simulink model "Airshow_hotpursuit_withadjustheight"  (R2012b)
settings: Solver=ode5  StartTime=0.0  StopTime=inf  FixedStep=sample_time  RelTol=1e-3
InitFcn:
  | sample_time=0.005;%0.004;%0.0025;%0.02;
  | sample_time_Vicon = 0.005;
  | DeltaT = 0.02;
  | g = 9.81;
  | H0 = g%0.3165;
  | Kl = 1;
  | 
  | Q6_mass = 0.84;
  | 
  | Q6_Omega_r = 1.5; %for horizon ref
  | Q6_Zeta_r = 0.5; %for horizon ref
  | Q6_Omega_r_h = 2;%for vertical ref
  | Q6_Zeta_r_h = 2; %for vertical ref
  | 
  | 
  | Q6_Omega = 1.5; %for horizon control
  | Q6_Zeta = 0.5; %for horizon control
  | Q6_Omega_h= 2; %for vertical control
  | Q6_Zeta_h = 0.7; %for vertical control
  | 
  | 
  | Q6_acc_max = 5;%horizontal max acc
  | Q6_acc_max_h = 3;%horizontal max acc
  | 
  | omega_circle = 72*pi/180;
  | omega_h = 0.1;%Ascending speed
  | PI = pi;
  | Circle_R = 2.5;
  | MAX_Height = -2;
undefined symbols (not defined in the file or in its folder): DiscIntNeverNeededParam
libraries: X330_Control x5, dspswit3 x5, simulink x4
(part 2 of 4)

== matlab function Airshow_hotpursuit_withadjustheight/UAV 1/Trajectory Logic/trackbounded1 ==
  data: cpx input; cpy input; region output; cvx input; cvy input; newx output; newy output; newregion output; estsecond input; chkfinalx output; chkfinaly output; chknum output; directionflag output; distanceall output; limitspeed input; cvxy output; time input; heightcontrol output
function [region,newx,newy,newregion,chkfinalx,chkfinaly,chknum,directionflag,distanceall,cvxy,heightcontrol]  = fcn(cpx,cpy,cvx,cvy,estsecond,limitspeed,time)
%#codegen
%cp = [cpy,cpx,0];
%cpest = [estrawy, estrawx,0];
%%database of check points
if(time<1)
    cvxy = 0;
else
cvxy = sqrt(cvx^2 + cvy^2);
end
chk0x = 3.239;
chk0y = 0.7037;
chk1x = 2.598;
chk1y = 1.13;
chk2x = 1.853;
chk2y = 1.266;
chk3x = 1.124;
chk3y = 1.462;
chk4x = 0.39;
chk4y = 1.935;
chk5x = -0.393;
chk5y = 2.012;
chk6x = -1.038;
chk6y = 1.521;
chk7x = -1.644;
chk7y = 1.023;
chk8x = -2.269;
chk8y = 1.058;
chk9x = -2.847;
chk9y = 1.469;
chk10x = -3.795;
chk10y = 1.337;
chk11x = -3.985;
chk11y = 0.42;
chk12x = -3.844;
chk12y = -0.55;
chk13x = -3.363;
chk13y = -1.263;
chk14x = -2.592;
chk14y = -1.786;
chk15x = -1.645;
chk15y = -2.067;
chk16x = -0.5438;
chk16y = -2.227;
chk17x = 0.425;
chk17y = -2.141;
chk18x = 1.192;
chk18y = -1.755;
chk19x = 2.025;
chk19y = -1.113;
chk20x = 3.12;
chk20y = -0.9148;
%%%%%%%%%%%%%%%%%%%%%%%%%%%%%%%%%%%%%%%%%%%%%%%%%%%%%%%%%%%
chk0 = [chk0y,chk0x,0];
chk1 = [chk1y,chk1x,0];
chk2 = [chk2y,chk2x,0];
chk3 = [chk3y,chk3x,0];
chk4 = [chk4y,chk4x,0];
chk5 = [chk5y,chk5x,0];
chk6 = [chk6y,chk6x,0];
chk7 = [chk7y,chk7x,0];
chk8 = [chk8y,chk8x,0];
chk9 = [chk9y,chk9x,0];
chk10 = [chk10y,chk10x,0];
chk11 = [chk11y,chk11x,0];
chk12 = [chk12y,chk12x,0];
chk13 = [chk13y,chk13x,0];
chk14 = [chk14y,chk14x,0];
chk15 = [chk15y,chk15x,0];
chk16 = [chk16y,chk16x,0];
chk17 = [chk17y,chk17x,0];
chk18 = [chk18y,chk18x,0];
chk19 = [chk19y,chk19x,0];
chk20 = [chk20y,chk20x,0];


distance01 = sqrt((chk0y-chk1y)^2+(chk0x-chk1x)^2);
distance12 = sqrt((chk2y-chk1y)^2+(chk2x-chk1x)^2);
distance23 = sqrt((chk2y-chk3y)^2+(chk2x-chk3x)^2);
distance34 = sqrt((chk3y-chk4y)^2+(chk3x-chk4x)^2);
distance45 = sqrt((chk4y-chk5y)^2+(chk4x-chk5x)^2);
distance56 = sqrt((chk5y-chk6y)^2+(chk5x-chk6x)^2);
distance67 = sqrt((chk6y-chk7y)^2+(chk6x-chk7x)^2);
distance78 = sqrt((chk7y-chk8y)^2+(chk7x-chk8x)^2);
distance89 = sqrt((chk8y-chk9y)^2+(chk8x-chk9x)^2);
distance910 = sqrt((chk9y-chk10y)^2+(chk9x-chk10x)^2);
distance1011 = sqrt((chk10y-chk11y)^2+(chk10x-chk11x)^2);
distance1112 = sqrt((chk11y-chk12y)^2+(chk11x-chk12x)^2);
distance1213 = sqrt((chk12y-chk13y)^2+(chk12x-chk13x)^2);
distance1314 = sqrt((chk13y-chk14y)^2+(chk13x-chk14x)^2);
distance1415 = sqrt((chk14y-chk15y)^2+(chk14x-chk15x)^2);
distance1516 = sqrt((chk15y-chk16y)^2+(chk15x-chk16x)^2);
distance1617 = sqrt((chk16y-chk17y)^2+(chk16x-chk17x)^2);
distance1718 = sqrt((chk17y-chk18y)^2+(chk17x-chk18x)^2);
distance1819 = sqrt((chk18y-chk19y)^2+(chk18x-chk19x)^2);
distance1920 = sqrt((chk19y-chk20y)^2+(chk19x-chk20x)^2);
distance200 = sqrt((chk20y-chk0y)^2+(chk20x-chk0x)^2);
distanceall = distance01 + distance12 + distance23+distance34+distance45+distance56+distance67+distance78+distance89+distance910+distance1011+distance1112+distance1213+distance1314+distance1415+distance1516+distance1617+distance1718+distance1819+distance1920+distance200;
%%%%%%%%%%%%%%%%%%%%%%%%%%%%%%%%%%%%%%%%%%%%%%%%%%%%%%%%%%%%%%%%%%%%%%%%%%%%%%%%%%%%%%region selector
if(cpx>-5 && cpx<=-4 && cpy>-3 && cpy<=-2)
    region = 0;
elseif(cpx>-4 && cpx<=-3 && cpy>-3 && cpy<=-2 )
    region = 1;
elseif(cpx>-3 && cpx<=-2 && cpy>-3 && cpy<=-2 )
    region = 2;
elseif(cpx>-2 && cpx<=-1 && cpy>-3 &&cpy<=-2)
    region = 3;
elseif(cpx>-1 && cpx<=0 && cpy>-3 && cpy<=-2)
    region = 4;
elseif(cpx>0 && cpx<=1 &&cpy>-3 && cpy<=-2)
    region = 5;
elseif(cpx>1 && cpx<=2 && cpy>-3 && cpy<=-2)
    region = 6;
elseif(cpx>2 && cpx<=3 && cpy>-3 && cpy<=-2)
    region = 7;
elseif(cpx>3 && cpx<=4 && cpy>-3 && cpy<=-2)
    region = 8;
elseif(cpx>4&& cpx<=5 && cpy>-3 && cpy<=-2)
    region = 9;
elseif(cpx>-5 && cpx<=-4 && cpy>-2 && cpy<=-1)
    region = 10;
elseif(cpx>-4 && cpx<=-3 && cpy>-2 && cpy<=-1)
    region = 11;
elseif(cpx>-3 && cpx<=-2 && cpy>-2 && cpy<=-1)
    region = 12;
elseif(cpx>-2 && cpx<=-1 && cpy>-2 && cpy<=-1)
    region = 13;
elseif(cpx>-1 && cpx<=0 && cpy>-2 && cpy<=-1)
    region = 14;
elseif(cpx>0 && cpx<=1 && cpy>-2 && cpy<=-1)
    region = 15;
elseif(cpx>1 && cpx<=2 && cpy>-2 && cpy<=-1)
    region = 16;
elseif(cpx>2 && cpx<=3 && cpy>-2 && cpy<=-1)
    region = 17;
elseif(cpx>3 && cpx<=4 && cpy>-2 && cpy<=-1)
    region = 18;
elseif(cpx>4 && cpx<=5 && cpy>-2 && cpy<=-1)
    region = 19;
elseif(cpx>-5 && cpx<=-4 && cpy>-1 && cpy<=0)
    region = 20;
elseif(cpx>-4 && cpx<=-3 && cpy>-1 && cpy<=0)
    region = 21;
elseif(cpx>-3 && cpx<=-2 && cpy>-1 && cpy<=0)
    region = 22;
elseif(cpx>-2 && cpx<=-1 && cpy>-1 && cpy<=0)
    region = 23;
elseif(cpx>-1 && cpx<=0 && cpy>-1 && cpy<=0)
    region = 24;
elseif(cpx>0 && cpx<=1 && cpy>-1 && cpy<=0)
    region = 25;
elseif(cpx>1 && cpx<=2 && cpy>-1 && cpy<=0)
    region = 26;
elseif(cpx>2 && cpx<=3 && cpy>-1 && cpy<=0)
    region = 27;
elseif(cpx>3 && cpx<=4 && cpy>-1 && cpy<=0)
    region = 28;
elseif(cpx>4 && cpx<=5 && cpy>-1 && cpy<=0)
    region = 29;
elseif(cpx>-5 && cpx<=-4 && cpy>0 && cpy<=1)
    region = 30;
elseif(cpx>-4 && cpx<=-3 && cpy>0 && cpy<=1)
    region = 31;
elseif(cpx>-3 && cpx<=-2 && cpy>0 && cpy<=1)
    region = 32;
elseif(cpx>-2 && cpx<=-1 && cpy>0 && cpy<=1)
    region = 33;
elseif(cpx>-1 && cpx<=0 && cpy>0 && cpy<=1)
    region = 34;
elseif(cpx>0 && cpx<=1 && cpy>0 && cpy<=1)
    region = 35;
elseif(cpx>1 && cpx<=2 && cpy>0 && cpy<=1)
    region = 36;
elseif(cpx>2 && cpx<=3 && cpy>0 && cpy<=1)
    region = 37;
elseif(cpx>3 && cpx<=4 && cpy>0 && cpy<=1)
    region = 38;
elseif(cpx>4 && cpx<=5 && cpy>0 && cpy<=1)
    region = 39;
elseif(cpx>-5 && cpx<=-4 && cpy>1 && cpy<=2)
    region = 40;
elseif(cpx>-4 && cpx<=-3 && cpy>1 && cpy<=2)
    region = 41;
elseif(cpx>-3 && cpx<=-2&& cpy>1 && cpy<=2)
    region = 42;
elseif(cpx>-2 && cpx<=-1 && cpy>1 && cpy<=2)
    region = 43;
elseif(cpx>-1 && cpx<=0 && cpy>1 && cpy<=2)
    region = 44;
elseif(cpx>0 && cpx<=1 && cpy>1 && cpy<=2)
    region = 45;
elseif(cpx>1 && cpx<=2 && cpy>1 && cpy<=2)
    region = 46;
elseif(cpx>2 && cpx<=3 && cpy>1 && cpy<=2)
    region = 47;
elseif(cpx>3 && cpx<=4 && cpy>1 && cpy<=2)
    region = 48;
elseif(cpx>4 && cpx<=5 && cpy>1 && cpy<=2)
    region = 49;
elseif(cpx>-5 && cpx<=-4 && cpy>2 && cpy<=3)
    region = 50;
elseif(cpx>-4 && cpx<=-3 && cpy>2 && cpy<=3)
    region = 51;
elseif(cpx>-3 && cpx<=-2 && cpy>2 && cpy<=3)
    region = 52;
elseif(cpx>-2 && cpx<=-1 && cpy>2 && cpy<=3)
    region = 53;
elseif(cpx>-1 && cpx<=0 && cpy>2 && cpy<=3)
    region = 54;
elseif(cpx>0 && cpx<=1 && cpy>2 && cpy<=3)
    region = 55;
elseif(cpx>1 && cpx<=2 && cpy>2 && cpy<=3)
    region = 56;
elseif(cpx>2 && cpx<=3 && cpy>2 && cpy<=3)
    region = 57;
elseif(cpx>3 && cpx<=4 && cpy>2 && cpy<=3)
    region = 58;
elseif(cpx>4 && cpx<=5 && cpy>2 && cpy<=3)
    region = 59;
else
    region = -1;
end
%%%%%%%%%%%%%%%%%%%%%%%%%%%%%%%%%%%%%%%%%%%%%%%%%%%%%%%%%%%%%%%%%%%%%%%%%%%%%%%%%%%%%%%%%%%%%%%%%%
if(region==37 ||region==48)
    %%%%%%%%%%%%%%%%calculate point to line distance%%%%%%%%%%%
    %a = chk1 - chk0;
   % b = cp - chk0;
    %d = norm(cross(a,b)) / norm(a);
    angle = atan2((chk1x-chk0x),(chk1y-chk0y));
    samplex = chk0x;
    sampley = chk0y;
    zero = 1;

elseif(region == 36||region==47)
    %a = chk2 - chk1;
   % b = cp - chk1;
   % d = norm(cross(a,b)) / norm(a);
    angle = atan2((chk2x-chk1x),(chk2y-chk1y));
    zero = 1;
    samplex = chk1x;
    sampley = chk1y;
elseif(region == 46 ||region==56)
    %a = chk3 - chk2;
    %b = cp - chk2;
   % d = norm(cross(a,b)) / norm(a);
    angle = atan2((chk3x-chk2x),(chk3y-chk2y));
    zero = 1;
    samplex = chk2x;
    sampley = chk2y;
elseif(region == 45 || region==55 ||region==35)
   % a = chk4 - chk3;
   % b = cp - chk3;
    %d = norm(cross(a,b)) / norm(a);
    angle = atan2((chk4x-chk3x),(chk4y-chk3y));
    zero = 1;
      samplex = chk3x;
    sampley = chk3y;
elseif(region == 54||region==44)
    %a = chk5 - chk4;
    %b = cp - chk4;
    %d = norm(cross(a,b)) / norm(a);
    angle = atan2((chk5x-chk4x),(chk5y-chk4y));
    zero = 1;
    samplex = chk4x;
    sampley = chk4y;
elseif(region == 43||region==53)
    %a = chk6 - chk5;
    %b = cp - chk5;
    %d = norm(cross(a,b)) / norm(a);
    angle = atan2((chk6x-chk5x),(chk6y-chk5y));
    zero = 1;
    samplex = chk5x;
    sampley = chk5y;
elseif(region==33||region==34)
    %a = chk7 - chk6;
    %b = cp - chk6;
    %d = norm(cross(a,b)) / norm(a);
    angle = atan2((chk7x-chk6x),(chk7y-chk6y));
    zero = 1;
    samplex = chk6x;
    sampley = chk6y;
elseif(region == 32)
    %a = chk8 - chk7;
    %b = cp - chk7;
    %d = norm(cross(a,b)) / norm(a);
    angle = atan2((chk8x-chk7x),(chk8y-chk7y));
    zero = 1;
    samplex = chk7x;
    sampley = chk7y;
elseif(region==42)
    %a = chk9 - chk8;
    %b = cp - chk8;
    %d = norm(cross(a,b)) / norm(a);
    angle = atan2((chk9x-chk8x),(chk9y-chk8y));
    zero = 1;
    samplex = chk8x;
    sampley = chk8y;
elseif(region == 41||region==31)
    %a = chk10 - chk9;
    %b = cp - chk9;
    %d = norm(cross(a,b)) / norm(a);
    angle = atan2((chk10x-chk9x),(chk10y-chk9y));
    zero = 1;
    samplex = chk9x;
    sampley = chk9y;
elseif(region == 30||region==40)
    %a = chk11 - chk10;
    %b = cp - chk10;
    %d = norm(cross(a,b)) / norm(a);
    angle = atan2((chk11x-chk10x),(chk11y-chk10y));
    zero = 1;
    samplex = chk10x;
    sampley = chk10y;
elseif(region == 20||region==21)
    %a = chk12 - chk11;
    %b = cp - chk11;
    %d = norm(cross(a,b)) / norm(a);
    angle = atan2((chk12x-chk11x),(chk12y-chk11y));
    zero = 1;
    samplex = chk11x;
    sampley = chk11y;
elseif(region == 10||region==11)
    %a = chk13 - chk12;
    %b = cp - chk12;
    %d = norm(cross(a,b)) / norm(a);
    angle = atan2((chk13x-chk12x),(chk13y-chk12y));
    zero = 1;
    samplex = chk12x;
    sampley = chk12y;
elseif(region == 1||region==12)
    %a = chk14 - chk13;
    %b = cp - chk13;
    %d = norm(cross(a,b)) / norm(a);
    angle = atan2((chk14x-chk13x),(chk14y-chk13y));
    zero = 1;
    samplex = chk13x;
    sampley = chk13y;
elseif(region == 2||region==13)
    %a = chk15 - chk14;
    %b = cp - chk14;
    %d = norm(cross(a,b)) / norm(a);
    angle = atan2((chk15x-chk14x),(chk15y-chk14y));
    zero = 1;
    samplex = chk14x;
    sampley = chk14y;
elseif(region == 3||region==14)
    %a = chk16 - chk15;
    %b = cp - chk15;
    %d = norm(cross(a,b)) / norm(a);
    angle = atan2((chk16x-chk15x),(chk16y-chk15y));
    zero = 1;
    samplex = chk15x;
    sampley = chk15y;
elseif(region == 4||region==5)
    %a = chk17 - chk16;
    %b = cp - chk16;
    %d = norm(cross(a,b)) / norm(a);
    angle = atan2((chk17x-chk16x),(chk17y-chk16y));
    zero = 1;
    samplex = chk16x;
    sampley = chk16y;
elseif(region == 6||region==15)
    %a = chk18 - chk17;
    %b = cp - chk17;
    %d = norm(cross(a,b)) / norm(a);
    angle = atan2((chk18x-chk17x),(chk18y-chk17y));
    zero = 1;
    samplex = chk17x;
    sampley = chk17y;
elseif(region == 16||region==7||region==25)
    %a = chk19 - chk18;
    %b = cp - chk18;
    %d = norm(cross(a,b)) / norm(a);
    angle = atan2((chk19x-chk18x),(chk19y-chk18y));
    zero = 1;
    samplex = chk18x;
    sampley = chk18y;
elseif(region == 26||region==27||region == 17 || region == 18)%%%%%%%%%%%%%%%%%%%%%%%%%%%%%%%%%%%%%%%%%%%%%%%%need to test
    %a = chk20 - chk19;
    %b = cp - chk19;
    %d = norm(cross(a,b)) / norm(a);
    angle = atan2((chk20x-chk19x),(chk20y-chk19y));
    zero = 1;
    samplex = chk19x;
    sampley = chk19y;
elseif(region == 28||region==29||region == 38 || region == 39) %%need to test 6 feb
    %a = chk0 - chk20;
    %b = cp - chk20;
    %d = norm(cross(a,b)) / norm(a);
    angle = atan2((chk0x-chk20x),(chk0y-chk20y));
    zero = 1;
    samplex = chk20x;
    sampley = chk20y;
else
    %a = -1;
   % b = -1;
    %d = -1;
    angle = -1;%%% i know this is not correct i will add one more zero coefficient to cancel this case
    zero = 0;
    samplex = 0;
    sampley = 0;
end


%%%%%%%%%%%%%%%%%%%%%%%%%%%%%%%%%%%%%%%%%%%%%%%%%%%%%%%%%%%%%%%%%%%%%%%%%%%%%%%%%%%%%%%%%%%%%%%%%%
% %%calculate project point on the check point line
if(zero == 0)%%if out of boundary none of the region match
        newy = 100;
        newx = 100;
else   %%match the region

        if(angle == 0 ||angle == 180)
            newx  = samplex;
            newy = cpy;
        elseif(angle == 90 || angle == 270)
            newx = cpx;
            newy = sampley;
        else
         kk = -1/(tan(angle));
         m = cpx - kk*cpy ;
         k = tan(angle);
         newy = (samplex - k*sampley - m)/(kk - k);
         newx = kk*newy + m;
         end

end

if(newx>-5 && newx<=-4 && newy>-3 && newy<=-2)
    newregion = 0;
elseif(newx>-4 && newx<=-3 && newy>-3 && newy<=-2 )
    newregion = 1;
elseif(newx>-3 && newx<=-2 && newy>-3 && newy<=-2 )
    newregion = 2;
elseif(newx>-2 && newx<=-1 && newy>-3 &&newy<=-2)
    newregion = 3;
elseif(newx>-1 && newx<=0 && newy>-3 && newy<=-2)
    newregion = 4;
elseif(newx>0 && newx<=1 &&newy>-3 && newy<=-2)
    newregion = 5;
elseif(newx>1 && newx<=2 && newy>-3 && newy<=-2)
    newregion = 6;
elseif(newx>2 && newx<=3 && newy>-3 && newy<=-2)
    newregion = 7;
elseif(newx>3 && newx<=4 && newy>-3 && newy<=-2)
    newregion = 8;
elseif(newx>4&& newx<=5 && newy>-3 && newy<=-2)
    newregion = 9;
elseif(newx>-5 && newx<=-4 && newy>-2 && newy<=-1)
    newregion = 10;
elseif(newx>-4 && newx<=-3 && newy>-2 && newy<=-1)
    newregion = 11;
elseif(newx>-3 && newx<=-2 && newy>-2 && newy<=-1)
    newregion = 12;
elseif(newx>-2 && newx<=-1 && newy>-2 && newy<=-1)
    newregion = 13;
elseif(newx>-1 && newx<=0 && newy>-2 && newy<=-1)
    newregion = 14;
elseif(newx>0 && newx<=1 && newy>-2 && newy<=-1)
    newregion = 15;
elseif(newx>1 && newx<=2 && newy>-2 && newy<=-1)
    newregion = 16;
elseif(newx>2 && newx<=3 && newy>-2 && newy<=-1)
    newregion = 17;
elseif(newx>3 && newx<=4 && newy>-2 && newy<=-1)
    newregion = 18;
elseif(newx>4 && newx<=5 && newy>-2 && newy<=-1)
    newregion = 19;
elseif(newx>-5 && newx<=-4 && newy>-1 && newy<=0)
    newregion = 20;
elseif(newx>-4 && newx<=-3 && newy>-1 && newy<=0)
    newregion = 21;
elseif(newx>-3 && newx<=-2 && newy>-1 && newy<=0)
    newregion = 22;
elseif(newx>-2 && newx<=-1 && newy>-1 && newy<=0)
    newregion = 23;
elseif(newx>-1 && newx<=0 && newy>-1 && newy<=0)
    newregion = 24;
elseif(newx>0 && newx<=1 && newy>-1 && newy<=0)
    newregion = 25;
elseif(newx>1 && newx<=2 && newy>-1 && newy<=0)
    newregion = 26;
elseif(newx>2 && newx<=3 && newy>-1 && newy<=0)
    newregion = 27;
elseif(newx>3 && newx<=4 && newy>-1 && newy<=0)
    newregion = 28;
elseif(newx>4 && newx<=5 && newy>-1 && newy<=0)
    newregion = 29;
elseif(newx>-5 && newx<=-4 && newy>0 && newy<=1)
    newregion = 30;
elseif(newx>-4 && newx<=-3 && newy>0 && newy<=1)
    newregion = 31;
elseif(newx>-3 && newx<=-2 && newy>0 && newy<=1)
    newregion = 32;
elseif(newx>-2 && newx<=-1 && newy>0 && newy<=1)
    newregion = 33;
elseif(newx>-1 && newx<=0 && newy>0 && newy<=1)
    newregion = 34;
elseif(newx>0 && newx<=1 && newy>0 && newy<=1)
    newregion = 35;
elseif(newx>1 && newx<=2 && newy>0 && newy<=1)
    newregion = 36;
elseif(newx>2 && newx<=3 && newy>0 && newy<=1)
    newregion = 37;
elseif(newx>3 && newx<=4 && newy>0 && newy<=1)
    newregion = 38;
elseif(newx>4 && newx<=5 && newy>0 && newy<=1)
    newregion = 39;
elseif(newx>-5 && newx<=-4 && newy>1 && newy<=2)
    newregion = 40;
elseif(newx>-4 && newx<=-3 && newy>1 && newy<=2)
    newregion = 41;
elseif(newx>-3 && newx<=-2&& newy>1 && newy<=2)
    newregion = 42;
elseif(newx>-2 && newx<=-1 && newy>1 && newy<=2)
    newregion = 43;
elseif(newx>-1 && newx<=0 && newy>1 && newy<=2)
    newregion = 44;
elseif(newx>0 && newx<=1 && newy>1 && newy<=2)
    newregion = 45;
elseif(newx>1 && newx<=2 && newy>1 && newy<=2)
    newregion = 46;
elseif(newx>2 && newx<=3 && newy>1 && newy<=2)
    newregion = 47;
elseif(newx>3 && newx<=4 && newy>1 && newy<=2)
    newregion = 48;
elseif(newx>4 && newx<=5 && newy>1 && newy<=2)
    newregion = 49;
elseif(newx>-5 && newx<=-4 && newy>2 && newy<=3)
    newregion = 50;
elseif(newx>-4 && newx<=-3 && newy>2 && newy<=3)
    newregion = 51;
elseif(newx>-3 && newx<=-2 && newy>2 && newy<=3)
    newregion = 52;
elseif(newx>-2 && newx<=-1 && newy>2 && newy<=3)
    newregion = 53;
elseif(newx>-1 && newx<=0 && newy>2 && newy<=3)
    newregion = 54;
elseif(newx>0 && newx<=1 && newy>2 && newy<=3)
    newregion = 55;
elseif(newx>1 && newx<=2 && newy>2 && newy<=3)
    newregion = 56;
elseif(newx>2 && newx<=3 && newy>2 && newy<=3)
    newregion = 57;
elseif(newx>3 && newx<=4 && newy>2 && newy<=3)
    newregion = 58;
elseif(newx>4 && newx<=5 && newy>2 && newy<=3)
    newregion = 59;
else
    newregion = -1;
end

%%%%%%%%%%%%%%%%%%%%%%%%%%%%%%%%%%%%%%%%%%%%%%%%%%%%%%%%%%%%%%%%%%%%%%%%%%%%
% if(posx>-2 && posx<=-1 && posy>1 && posy<=2)
%     posregion = 0;
% elseif(posx>-1 && posx<=0 && posy>1 && posy<=2 )
%     posregion = 1;
% elseif(posx>0 && posx<=1 && posy>1 && posy<=2 )
%     posregion = 2;
% elseif(posx>-2 && posx<=-1 && posy>0 &&posy<=1)
%     posregion = 3;
% elseif(posx>-1 && posx<=0 && posy>0 && posy<=1)
%     posregion = 4;
% elseif(posx>-2 && posx<=-1 &&posy>-1 && posy<=0)
%     posregion = 5;
% elseif(posx>-1 && posx<=0 && posy>-1 && posy<=0)
%     posregion = 6;
% elseif(posx>-2 && posx<=-1 && posy>-2 && posy<=-1)
%     posregion = 7;
% elseif(posx>-1 && posx<=0 && posy>-2 && posy<=-1)
%     posregion = 8;
% elseif(posx>0 && posx<=1 && posy>-2 && posy<=-1)
%     posregion = 9;
% elseif(posx>1 && posx<=2 && posy>-2 && posy<=-1)
%     posregion = 10;
% elseif(posx>0 && posx<=1 && posy>-1 && posy<=0)
%     posregion = 11;
% elseif(posx>1 && posx<=2 && posy>-1 && posy<=0)
%     posregion = 12;
% elseif(posx>1 && posx<=2 && posy>0 && posy<=1)
%     posregion = 13;
% elseif(posx>1 && posx<=2 && posy>1 && posy<=2)
%     posregion = 14;
% elseif(posx>0 && posx<=1 && posy>0 && posy<=1)
%     posregion = 15;
% elseif(posx>2 && posx<=3 && posy>-2 && posy<=-1)
%     posregion = 16;
% elseif(posx>1 && posx<=2 && posy>-3 && posy<=-2)
%     posregion = 17;
% elseif(posx>2 && posx<=3 && posy>-3 && posy<=-2)
%     posregion = 18;
% elseif(posx>0 && posx<=1 && posy>-3 && posy<=-2)
%     posregion = 19;
% elseif(posx>-1 && posx<=0 && posy>-3 && posy<=-2)
%     posregion = 20;
% elseif(posx>2 && posx<=3 && posy>-1 && posy<=0)
%     posregion = 21;
% elseif(posx>2 && posx<=3 && posy>0 && posy<=1)
%     posregion = 22;
% elseif(posx>1 && posx<=2 && posy>2 && posy<=3)
%     posregion = 23;
% elseif(posx>0 && posx<=1 && posy>2 && posy<=3)
%    posregion = 24;
% elseif(posx>-1 && posx<=0 && posy>2 && posy<=3)
%     posregion = 25;
% else
%     posregion = -1;
% end


%%%%%%%%%%%%%%%%%%%%%%%%%%%%%%%%%%%%%%%%%%%%%%%%%%%%%%%%%%%%%%%%%%%%%%%%%
velangle = atan2(cvx,cvy);
diffvelangletoangle = velangle - angle;
velproject = (cvx^2 + cvy^2)*cos(diffvelangletoangle);
estdistance = estsecond * velproject;
vxyM = sqrt(cvx^2 + cvy^2);
cosdiffvelangletoangle = cos(diffvelangletoangle);
if(vxyM < limitspeed)
    directionflag = 0;
    %frontbackflag = -1;
    %diffuavcartoangle = -9999;
else
if(cosdiffvelangletoangle>=0)
    directionflag = 1;
else
    directionflag = -1;
end
%uavcarvectorangle = atan2((posx-newx),(posy-newy));
%diffuavcartoangle = uavcarvectorangle - angle;
% cosdiffuavcartoangle = cos(diffuavcartoangle);
% if(cosdiffuavcartoangle>=0)
%     frontbackflag = 1;
% else
%     frontbackflag = 0;
% end
end
%if(directionflag == 1)
if(newregion == 48 ||newregion==37)
    newdistancetonext = sqrt((newy-chk1y)^2+(newx-chk1x)^2);
    if(estdistance < (newdistancetonext))
        chkfinalx = chk1x;
        chkfinaly = chk1y;
        chknum = 1;
    elseif(estdistance>=(newdistancetonext) && estdistance <((newdistancetonext) + distance12))
        chkfinalx = chk2x;
        chkfinaly = chk2y;
        chknum = 2;
    elseif(estdistance>=((newdistancetonext)+distance12)&&estdistance<((newdistancetonext)+distance12+distance23))
        chkfinalx = chk3x;
        chkfinaly = chk3y;
        chknum = 3;
    elseif(estdistance>=((newdistancetonext)+distance12+distance23)&&estdistance<((newdistancetonext)+distance12+distance23+distance34))
        chkfinalx = chk4x;
        chkfinaly = chk4y;
        chknum = 4;
    elseif(estdistance>=((newdistancetonext)+distance12+distance23+distance34)&&estdistance<((newdistancetonext)+distance12+distance23+distance34+distance45))
        chkfinalx = chk5x;
        chkfinaly = chk5y;
        chknum = 5;
    else
        chkfinalx = chk5x;
        chkfinaly = chk5y;
        chknum = 5;
    end
elseif(newregion == 36||newregion==47)
    newdistancetonext = sqrt((newy-chk2y)^2+(newx-chk2x)^2);
    if(estdistance < (newdistancetonext))
        chkfinalx = chk2x;
        chkfinaly = chk2y;
        chknum = 2;
    elseif(estdistance >=(newdistancetonext)&&estdistance < ((newdistancetonext)+distance23))
        chkfinalx = chk3x;
        chkfinaly = chk3y;
        chknum = 3;
    elseif(estdistance >=((newdistancetonext)+distance23)&&estdistance < ((newdistancetonext)+distance23+distance34))
        chkfinalx = chk4x;
        chkfinaly = chk4y;
        chknum = 4;
    elseif(estdistance >=((newdistancetonext)+distance23+distance34)&&estdistance < ((newdistancetonext)+distance23+distance34+distance45))
        chkfinalx = chk5x;
        chkfinaly = chk5y;
        chknum = 5;
    elseif(estdistance >=((newdistancetonext)+distance23+distance34+distance45)&&estdistance < ((newdistancetonext)+distance23+distance34+distance45+distance56))
        chkfinalx = chk6x;
        chkfinaly = chk6y;
        chknum = 6;
    else
        chkfinalx = chk6x;
        chkfinaly = chk6y;
        chknum = 6;
    end
elseif(newregion == 46||newregion==56)
    newdistancetonext = sqrt((newy-chk3y)^2+(newx-chk3x)^2);
    if(estdistance < (newdistancetonext))
        chkfinalx = chk3x;
        chkfinaly = chk3y;
        chknum = 3;
    elseif((estdistance >= (newdistancetonext))&&estdistance<((newdistancetonext)+distance34))
        chkfinalx = chk4x;
        chkfinaly = chk4y;
        chknum = 4;
    elseif((estdistance >= (newdistancetonext)+distance34)&&estdistance<((newdistancetonext)+distance34+distance45))
        chkfinalx = chk5x;
        chkfinaly = chk5y;
        chknum = 5;
    elseif((estdistance >= (newdistancetonext)+distance34+distance45)&&estdistance<((newdistancetonext)+distance34+distance45+distance56))
        chkfinalx = chk6x;
        chkfinaly = chk6y;
        chknum = 6;
    elseif((estdistance >= (newdistancetonext)+distance34+distance45+distance56)&&estdistance<((newdistancetonext)+distance34+distance45+distance56+distance67))
        chkfinalx = chk7x;
        chkfinaly = chk7y;
        chknum = 7;
    else
        chkfinalx = chk7x;
        chkfinaly = chk7y;
        chknum = 7;
    end
elseif(newregion ==45 || newregion == 55|| newregion == 35)
    newdistancetonext = sqrt((newy-chk4y)^2+(newx-chk4x)^2);
    if(estdistance < (newdistancetonext))
        chkfinalx = chk4x;
        chkfinaly = chk4y;
        chknum = 4;
    elseif((estdistance >= (newdistancetonext))&&estdistance<((newdistancetonext)+distance45))
        chkfinalx = chk5x;
        chkfinaly = chk5y;
        chknum = 5;
    elseif((estdistance >= (newdistancetonext)+distance45)&&estdistance<((newdistancetonext)+distance45+distance56))
        chkfinalx = chk6x;
        chkfinaly = chk6y;
        chknum = 6;
    elseif((estdistance >= (newdistancetonext)+distance45+distance56)&&estdistance<((newdistancetonext)+distance45+distance56+distance67))
        chkfinalx = chk7x;
        chkfinaly = chk7y;
        chknum = 7;
    elseif((estdistance >= (newdistancetonext)+distance45+distance56+distance67)&&estdistance<((newdistancetonext)+distance45+distance56+distance67+distance78))
        chkfinalx = chk8x;
        chkfinaly = chk8y;
        chknum = 8;
    else
        chkfinalx = chk8x;
        chkfinaly = chk8y;
        chknum = 8;
    end
elseif(newregion == 54|| newregion == 44)
    newdistancetonext = sqrt((newy-chk5y)^2+(newx-chk5x)^2);
    if(estdistance < (newdistancetonext))
        chkfinalx = chk5x;
        chkfinaly = chk5y;
        chknum = 5;
    elseif((estdistance >= (newdistancetonext))&&estdistance<((newdistancetonext)+distance56))
        chkfinalx = chk6x;
        chkfinaly = chk6y;
        chknum = 6;
    elseif((estdistance >= (newdistancetonext)+distance56)&&estdistance<((newdistancetonext)+distance56+distance67))
        chkfinalx = chk7x;
        chkfinaly = chk7y;
        chknum = 7;
    elseif((estdistance >= (newdistancetonext)+distance56+distance67)&&estdistance<((newdistancetonext)+distance56+distance67+distance78))
        chkfinalx = chk8x;
        chkfinaly = chk8y;
        chknum = 8;
    elseif((estdistance >= (newdistancetonext)+distance56+distance67+distance78)&&estdistance<((newdistancetonext)+distance56+distance67+distance78+distance89))
        chkfinalx = chk9x;
        chkfinaly = chk9y;
        chknum = 9;
    else
        chkfinalx = chk9x;
        chkfinaly = chk9y;
        chknum = 9;
    end
elseif(newregion == 43|| newregion == 53)
    newdistancetonext = sqrt((newy-chk6y)^2+(newx-chk6x)^2);
    if(estdistance < (newdistancetonext))
        chkfinalx = chk6x;
        chkfinaly = chk6y;
        chknum = 6;
    elseif((estdistance >= (newdistancetonext))&&estdistance<((newdistancetonext)+distance67))
        chkfinalx = chk7x;
        chkfinaly = chk7y;
        chknum = 7;
    elseif((estdistance >= (newdistancetonext)+distance67)&&estdistance<((newdistancetonext)+distance67+distance78))
        chkfinalx = chk8x;
        chkfinaly = chk8y;
        chknum = 8;
    elseif((estdistance >= (newdistancetonext)+distance67+distance78)&&estdistance<((newdistancetonext)+distance67+distance78+distance89))
        chkfinalx = chk9x;
        chkfinaly = chk9y;
        chknum = 9;
    elseif((estdistance >= (newdistancetonext)+distance67+distance78+distance89)&&estdistance<((newdistancetonext)+distance67+distance78+distance89+distance910))
        chkfinalx = chk10x;
        chkfinaly = chk10y;
        chknum = 10;
    else
        chkfinalx = chk10x;
        chkfinaly = chk10y;
        chknum = 10;
    end
elseif(newregion == 33|| newregion == 34)
    newdistancetonext = sqrt((newy-chk7y)^2+(newx-chk7x)^2);
    if(estdistance < (newdistancetonext))
        chkfinalx = chk7x;
        chkfinaly = chk7y;
        chknum = 7;
    elseif((estdistance >= (newdistancetonext))&&estdistance<((newdistancetonext)+distance78))
        chkfinalx = chk8x;
        chkfinaly = chk8y;
        chknum = 8;
    elseif((estdistance >= (newdistancetonext)+distance78)&&estdistance<((newdistancetonext)+distance78+distance89))
        chkfinalx = chk9x;
        chkfinaly = chk9y;
        chknum = 9;
    elseif((estdistance >= (newdistancetonext)+distance78+distance89)&&estdistance<((newdistancetonext)+distance78+distance89+distance910))
        chkfinalx = chk10x;
        chkfinaly = chk10y;
        chknum = 10;
    elseif((estdistance >= (newdistancetonext)+distance78+distance89+distance910)&&estdistance<((newdistancetonext)+distance78+distance89+distance910+distance1011))
        chkfinalx = chk11x;
        chkfinaly = chk11y;
        chknum = 11;
    else
        chkfinalx = chk11x;
        chkfinaly = chk11y;
        chknum = 11;
    end
elseif(newregion == 32)
    newdistancetonext = sqrt((newy-chk8y)^2+(newx-chk8x)^2);
    if(estdistance < (newdistancetonext))
        chkfinalx = chk8x;
        chkfinaly = chk8y;
        chknum = 8;
    elseif((estdistance >= (newdistancetonext))&&estdistance<((newdistancetonext)+distance89))
        chkfinalx = chk9x;
        chkfinaly = chk9y;
        chknum = 9;
    elseif((estdistance >= (newdistancetonext)+distance89)&&estdistance<((newdistancetonext)+distance89+distance910))
        chkfinalx = chk10x;
        chkfinaly = chk10y;
        chknum = 10;
     elseif((estdistance >= (newdistancetonext)+distance89+distance910)&&estdistance<((newdistancetonext)+distance89+distance910+distance1011))
        chkfinalx = chk11x;
        chkfinaly = chk11y;
        chknum = 11;
%     elseif((estdistance >= (newdistancetonext)+distance89+distance910+distance1011)&&estdistance<((newdistancetonext)+distance89+distance910+distance1011+distance1112))
%         chkfinalx = chk12x;
%         chkfinaly = chk12y;
%         chknum = 12;
    else
        chkfinalx = chk11x;
        chkfinaly = chk11y;
        chknum = 11;
    end
elseif(newregion==42)
    newdistancetonext = sqrt((newy-chk9y)^2+(newx-chk9x)^2);
    if(estdistance < (newdistancetonext))
        chkfinalx = chk9x;
        chkfinaly = chk9y;
        chknum = 9;
    elseif((estdistance >= (newdistancetonext))&&estdistance<((newdistancetonext)+distance910))
        chkfinalx = chk10x;
        chkfinaly = chk10y;
        chknum = 10;
    elseif((estdistance >= (newdistancetonext)+distance910)&&estdistance<((newdistancetonext)+distance910+distance1011))
        chkfinalx = chk11x;
        chkfinaly = chk11y;
        chknum = 11;
    elseif((estdistance >= (newdistancetonext)+distance910+distance1011)&&estdistance<((newdistancetonext)+distance910+distance1011+distance1112))
        chkfinalx = chk12x;
        chkfinaly = chk12y;
        chknum = 12;
%     elseif((estdistance >= (newdistancetonext)+distance910+distance1011+distance1112)&&estdistance<((newdistancetonext)+distance910+distance1011+distance1112+distance1213))
%         chkfinalx = chk13x;
%         chkfinaly = chk13y;
%         chknum = 13;
    else
        chkfinalx = chk12x;
        chkfinaly = chk12y;
        chknum = 12;
    end
elseif(newregion == 41 || newregion == 31)
    newdistancetonext = sqrt((newy-chk10y)^2+(newx-chk10x)^2);
    if(estdistance < (newdistancetonext))
        chkfinalx = chk10x;
        chkfinaly = chk10y;
        chknum = 10;
    elseif((estdistance >= (newdistancetonext))&&estdistance<((newdistancetonext)+distance1011))
        chkfinalx = chk11x;
        chkfinaly = chk11y;
        chknum = 11;
    elseif((estdistance >= (newdistancetonext)+distance1011)&&estdistance<((newdistancetonext)+distance1011+distance1112))
        chkfinalx = chk12x;
        chkfinaly = chk12y;
        chknum = 12;
    elseif((estdistance >= (newdistancetonext)+distance1011+distance1112)&&estdistance<((newdistancetonext)+distance1011+distance1112+distance1213))
        chkfinalx = chk13x;
        chkfinaly = chk13y;
        chknum = 13;
    elseif((estdistance >= (newdistancetonext)+distance1011+distance1112+distance1213)&&estdistance<((newdistancetonext)+distance1011+distance1112+distance1213+distance1314))
        chkfinalx = chk14x;
        chkfinaly = chk14y;
        chknum = 14;
    else
        chkfinalx = chk14x;
        chkfinaly = chk14y;
        chknum = 14;
    end
elseif(newregion == 30 || newregion == 40)
    newdistancetonext = sqrt((newy-chk11y)^2+(newx-chk11x)^2);
    if(estdistance < (newdistancetonext))
        chkfinalx = chk11x;
        chkfinaly = chk11y;
        chknum = 11;
    elseif((estdistance >= (newdistancetonext))&&estdistance<((newdistancetonext)+distance1112))
        chkfinalx = chk12x;
        chkfinaly = chk12y;
        chknum = 12;
    elseif((estdistance >= (newdistancetonext)+distance1112)&&estdistance<((newdistancetonext)+distance1112+distance1213))
        chkfinalx = chk13x;
        chkfinaly = chk13y;
        chknum = 13;
    elseif((estdistance >= (newdistancetonext)+distance1112+distance1213)&&estdistance<((newdistancetonext)+distance1112+distance1213+distance1314))
        chkfinalx = chk14x;
        chkfinaly = chk14y;
        chknum = 14;
    elseif((estdistance >= (newdistancetonext)+distance1112+distance1213+distance1314)&&estdistance<((newdistancetonext)+distance1112+distance1213+distance1314+distance1415))
        chkfinalx = chk15x;
        chkfinaly = chk15y;
        chknum = 15;
    else
        chkfinalx = chk15x;
        chkfinaly = chk15y;
        chknum = 15;
    end
elseif(newregion == 20|| newregion == 21)
    newdistancetonext = sqrt((newy-chk12y)^2+(newx-chk12x)^2);
    if(estdistance < (newdistancetonext))
        chkfinalx = chk12x;
        chkfinaly = chk12y;
        chknum = 12;
    elseif((estdistance >= (newdistancetonext))&&estdistance<((newdistancetonext)+distance1213))
        chkfinalx = chk13x;
        chkfinaly = chk13y;
        chknum = 13;
    elseif((estdistance >= (newdistancetonext)+distance1213)&&estdistance<((newdistancetonext)+distance1213+distance1314))
        chkfinalx = chk14x;
        chkfinaly = chk14y;
        chknum = 14;
    elseif((estdistance >= (newdistancetonext)+distance1213+distance1314)&&estdistance<((newdistancetonext)+distance1213+distance1314+distance1415))
        chkfinalx = chk15x;
        chkfinaly = chk15y;
        chknum = 15;
    elseif((estdistance >= (newdistancetonext)+distance1213+distance1314+distance1415)&&estdistance<((newdistancetonext)+distance1213+distance1314+distance1415+distance1516))
        chkfinalx = chk16x;
        chkfinaly = chk16y;
        chknum = 16;
    else
        chkfinalx = chk16x;
        chkfinaly = chk16y;
        chknum = 16;
    end
elseif(newregion == 10 || newregion == 11)
    newdistancetonext = sqrt((newy-chk13y)^2+(newx-chk13x)^2);
    if(estdistance < (newdistancetonext))
        chkfinalx = chk13x;
        chkfinaly = chk13y;
        chknum = 13;
    elseif((estdistance >= (newdistancetonext))&&estdistance<((newdistancetonext)+distance1314))
        chkfinalx = chk14x;
        chkfinaly = chk14y;
        chknum = 14;
    elseif((estdistance >= (newdistancetonext)+distance1314)&&estdistance<((newdistancetonext)+distance1314+distance1415))
        chkfinalx = chk15x;
        chkfinaly = chk15y;
        chknum = 15;
    elseif((estdistance >= (newdistancetonext)+distance1314+distance1415)&&estdistance<((newdistancetonext)+distance1314+distance1415+distance1516))
        chkfinalx = chk16x;
        chkfinaly = chk16y;
        chknum = 16;
    elseif((estdistance >= (newdistancetonext)+distance1314+distance1415+distance1516)&&estdistance<((newdistancetonext)+distance1314+distance1415+distance1516+distance1617))
        chkfinalx = chk17x;
        chkfinaly = chk17y;
        chknum = 17;
    else
        chkfinalx = chk17x;
        chkfinaly = chk17y;
        chknum = 17;
    end
elseif(newregion == 1|| newregion == 12)
    newdistancetonext = sqrt((newy-chk14y)^2+(newx-chk14x)^2);
    if(estdistance < (newdistancetonext))
        chkfinalx = chk14x;
        chkfinaly = chk14y;
        chknum = 14;
    elseif((estdistance >= (newdistancetonext))&&estdistance<((newdistancetonext)+distance1415))
        chkfinalx = chk15x;
        chkfinaly = chk15y;
        chknum = 15;
    elseif((estdistance >= (newdistancetonext)+distance1415)&&estdistance<((newdistancetonext)+distance1415+distance1516))
        chkfinalx = chk16x;
        chkfinaly = chk16y;
        chknum = 16;
    elseif((estdistance >= (newdistancetonext)+distance1415+distance1516)&&estdistance<((newdistancetonext)+distance1415+distance1516+distance1617))
        chkfinalx = chk17x;
        chkfinaly = chk17y;
        chknum = 17;
    elseif((estdistance >= (newdistancetonext)+distance1415+distance1516+distance1617)&&estdistance<((newdistancetonext)+distance1415+distance1516+distance1617+distance1718))
        chkfinalx = chk18x;
        chkfinaly = chk18y;
        chknum = 18;
    else
        chkfinalx = chk18x;
        chkfinaly = chk18y;
        chknum = 18;
    end
elseif(newregion == 13|| newregion == 2)
    newdistancetonext = sqrt((newy-chk15y)^2+(newx-chk15x)^2);
    if(estdistance < (newdistancetonext))
        chkfinalx = chk15x;
        chkfinaly = chk15y;
        chknum = 15;
    elseif((estdistance >= (newdistancetonext))&&estdistance<((newdistancetonext)+distance1516))
        chkfinalx = chk16x;
        chkfinaly = chk16y;
        chknum = 16;
    elseif((estdistance >= (newdistancetonext)+distance1516)&&estdistance<((newdistancetonext)+distance1516+distance1617))
        chkfinalx = chk17x;
        chkfinaly = chk17y;
        chknum = 17;
    elseif((estdistance >= (newdistancetonext)+distance1516+distance1617)&&estdistance<((newdistancetonext)+distance1516+distance1617+distance1718))
        chkfinalx = chk18x;
        chkfinaly = chk18y;
        chknum = 18;
    elseif((estdistance >= (newdistancetonext)+distance1516+distance1617+distance1718)&&estdistance<((newdistancetonext)+distance1516+distance1617+distance1718+distance1819))
        chkfinalx = chk19x;
        chkfinaly = chk19y;
        chknum = 19;
    else
        chkfinalx = chk19x;
        chkfinaly = chk19y;
        chknum = 19;
    end
elseif(newregion == 3|| newregion == 14)
    newdistancetonext = sqrt((newy-chk16y)^2+(newx-chk16x)^2);
    if(estdistance < (newdistancetonext))
        chkfinalx = chk16x;
        chkfinaly = chk16y;
        chknum = 16;
    elseif((estdistance >= (newdistancetonext))&&estdistance<((newdistancetonext)+distance1617))
        chkfinalx = chk17x;
        chkfinaly = chk17y;
        chknum = 17;
    elseif((estdistance >= (newdistancetonext)+distance1617)&&estdistance<((newdistancetonext)+distance1617+distance1718))
        chkfinalx = chk18x;
        chkfinaly = chk18y;
        chknum = 18;
    elseif((estdistance >= (newdistancetonext)+distance1617+distance1718)&&estdistance<((newdistancetonext)+distance1617+distance1718+distance1819))
        chkfinalx = chk19x;
        chkfinaly = chk19y;
        chknum = 19;
    elseif((estdistance >= (newdistancetonext)+distance1617+distance1718+distance1819)&&estdistance<((newdistancetonext)+distance1617+distance1718+distance1819+distance1920))
        chkfinalx = chk20x;
        chkfinaly = chk20y;
        chknum = 20;
    else
        chkfinalx = chk20x;
        chkfinaly = chk20y;
        chknum = 20;
    end
elseif(newregion == 4 || newregion == 5)
    newdistancetonext = sqrt((newy-chk17y)^2+(newx-chk17x)^2);
    if(estdistance < (newdistancetonext))
        chkfinalx = chk17x;
        chkfinaly = chk17y;
        chknum = 17;
    elseif((estdistance >= (newdistancetonext))&&estdistance<((newdistancetonext)+distance1718))
        chkfinalx = chk18x;
        chkfinaly = chk18y;
        chknum = 18;
    elseif((estdistance >= (newdistancetonext)+distance1718)&&estdistance<((newdistancetonext)+distance1718+distance1819))
        chkfinalx = chk19x;
        chkfinaly = chk19y;
        chknum = 19;
    elseif((estdistance >= (newdistancetonext)+distance1718+distance1819)&&estdistance<((newdistancetonext)+distance1718+distance1819+distance1920))
        chkfinalx = chk20x;
        chkfinaly = chk20y;
        chknum = 20;
%     elseif((estdistance >= (newdistancetonext)+distance1718+distance1819+distance1920)&&estdistance<((newdistancetonext)+distance1718+distance1819+distance1920+distance200))
%         chkfinalx = chk0x;
%         chkfinaly = chk0y;
%         chknum = 0;
    else
        chkfinalx = chk20x;
        chkfinaly = chk20y;
        chknum = 20;
    end
elseif(newregion == 6|| newregion == 15)
    newdistancetonext = sqrt((newy-chk18y)^2+(newx-chk18x)^2);
    if(estdistance < (newdistancetonext))
        chkfinalx = chk18x;
        chkfinaly = chk18y;
        chknum = 18;
    elseif((estdistance >= (newdistancetonext))&&estdistance<((newdistancetonext)+distance1819))
        chkfinalx = chk19x;
        chkfinaly = chk19y;
        chknum = 19;
    elseif((estdistance >= (newdistancetonext)+distance1819)&&estdistance<((newdistancetonext)+distance1819+distance1920))
        chkfinalx = chk20x;
        chkfinaly = chk20y;
        chknum = 20;
    elseif((estdistance >= (newdistancetonext)+distance1819+distance1920)&&estdistance<((newdistancetonext)+distance1819+distance1920+distance200))
        chkfinalx = chk0x;
        chkfinaly = chk0y;
        chknum = 0;
%     elseif((estdistance >= (newdistancetonext)+distance1819+distance1920+distance200)&&estdistance<((newdistancetonext)+distance1819+distance1920+distance200+distance01))
%         chkfinalx = chk1x;
%         chkfinaly = chk1y;
%         chknum = 1;
    else
        chkfinalx = chk0x;
        chkfinaly = chk0y;
        chknum = 0;
    end
elseif(newregion == 16|| newregion == 7|| newregion == 25)
    newdistancetonext = sqrt((newy-chk19y)^2+(newx-chk19x)^2);
    if(estdistance < (newdistancetonext))
        chkfinalx = chk19x;
        chkfinaly = chk19y;
        chknum = 19;
    elseif((estdistance >= (newdistancetonext))&&estdistance<((newdistancetonext)+distance1920))
        chkfinalx = chk20x;
        chkfinaly = chk20y;
        chknum = 20;
    elseif((estdistance >= (newdistancetonext)+distance1920)&&estdistance<((newdistancetonext)+distance1920+distance200))
        chkfinalx = chk0x;
        chkfinaly = chk0y;
        chknum = 0;
%     elseif((estdistance >= (newdistancetonext)+distance1920+distance200)&&estdistance<((newdistancetonext)+distance1920+distance200+distance01))
%         chkfinalx = chk1x;
%         chkfinaly = chk1y;
%         chknum = 1;
%     elseif((estdistance >= (newdistancetonext)+distance1920+distance200+distance01)&&estdistance<((newdistancetonext)+distance1920+distance200+distance01+distance12))
%         chkfinalx = chk2x;
%         chkfinaly = chk2y;
%         chknum = 2;
    else
        chkfinalx = chk0x;
        chkfinaly = chk0y;
        chknum = 0;
    end
elseif(newregion == 26 || newregion == 27||newregion == 17 || newregion==18)%%need to change
    newdistancetonext = sqrt((newy-chk20y)^2+(newx-chk20x)^2);
    if(estdistance < (newdistancetonext))
        chkfinalx = chk20x;
        chkfinaly = chk20y;
        chknum = 20;
    elseif((estdistance >= (newdistancetonext))&&estdistance<((newdistancetonext)+distance200))
        chkfinalx = chk0x;
        chkfinaly = chk0y;
        chknum = 0;
%     elseif((estdistance >= (newdistancetonext)+distance200)&&estdistance<((newdistancetonext)+distance200+distance01))
%         chkfinalx = chk1x;
%         chkfinaly = chk1y;
%         chknum = 1;
%     elseif((estdistance >= (newdistancetonext)+distance200+distance01)&&estdistance<((newdistancetonext)+distance200+distance01+distance12))
%         chkfinalx = chk2x;
%         chkfinaly = chk2y;
%         chknum = 2;
%     elseif((estdistance >= (newdistancetonext)+distance200+distance01+distance12)&&estdistance<((newdistancetonext)+distance200+distance01+distance12+distance23))
%         chkfinalx = chk3x;
%         chkfinaly = chk3y;
%         chknum = 3;
    else
        chkfinalx = chk0x;
        chkfinaly = chk0y;
        chknum = 0;
    end
    
elseif(newregion == 28 || newregion == 29||newregion==38||newregion==39) %%%%%%%%%%%need to change
    newdistancetonext = sqrt((newy-chk0y)^2+(newx-chk0x)^2);
    if(estdistance < (newdistancetonext))
        chkfinalx = chk0x;
        chkfinaly = chk0y;
        chknum = 0;
    elseif((estdistance >= (newdistancetonext))&&estdistance<((newdistancetonext)+distance01))
        chkfinalx = chk1x;
        chkfinaly = chk1y;
        chknum = 1;
%     elseif((estdistance >= (newdistancetonext)+distance01)&&estdistance<((newdistancetonext)+distance01+distance12))
%         chkfinalx = chk2x;
%         chkfinaly = chk2y;
%         chknum = 2;
%     elseif((estdistance >= (newdistancetonext)+distance01+distance12)&&estdistance<((newdistancetonext)+distance01+distance12+distance23))
%         chkfinalx = chk3x;
%         chkfinaly = chk3y;
%         chknum = 3;
%     elseif((estdistance >= (newdistancetonext)+distance01+distance12+distance23)&&estdistance<((newdistancetonext)+distance01+distance12+distance23+distance34))
%         chkfinalx = chk4x;
%         chkfinaly = chk4y;
%         chknum = 4;
    else
        chkfinalx = chk1x;
        chkfinaly = chk1y;
        chknum = 1;
    end
else
    newdistancetonext = -1;
    chkfinalx = 0;
    chkfinaly = 0;
    chknum = -1;
    
end
% elseif(directionflag==-1)
%        if()
% else
%            
% end
if((chknum >=0 && chknum<=10)||(chknum>=17 && chknum<=20))
    heightcontrol = 0;
elseif(chknum>=11 && chknum <=16)
   heightcontrol = -0.03;
else
   heightcontrol = 0;
end



%end

== matlab function Airshow_hotpursuit_withadjustheight/UAV 1/Trajectory Logic/wp_limit ==
  data: posdesiredx input; posdesiredy input; distancelimit input; posx input; posy input; newposdesiredx output; newposdesiredy output; smooth_flag input
function [newposdesiredx,newposdesiredy] = fcn(posdesiredx,posdesiredy,distancelimit,posx,posy,smooth_flag)
%#codegen
w = atan2((posdesiredx-posx),(posdesiredy-posy));
desiredtopos = sqrt((posdesiredy-posy)^2+(posdesiredx-posx)^2);
if(smooth_flag == 1)
    newposdesiredx = posdesiredx;
    newposdesiredy = posdesiredy;
    %newposdesiredx = posx + smoothdistancelimit*sin(w);
    %newposdesiredy = posy + smoothdistancelimit*cos(w);
else
if(desiredtopos <= distancelimit)
    newposdesiredx = posdesiredx;
    newposdesiredy = posdesiredy;
else
    newposdesiredx = posx + distancelimit*sin(w);
    newposdesiredy = posy + distancelimit*cos(w);
end
end
